simulink model "coursework"  (R2024a)
settings: Solver=FixedStepAuto  StartTime=0.0  StopTime=0.5  FixedStep=0.00001  RelTol=1e-3
values from neighbouring files (symbols this model uses):
  a1 = 80    [PMSM_parameters.m]
  a2 = 200    [PMSM_parameters.m]
  a3 = 360    [PMSM_parameters.m]
  a4 = 520    [PMSM_parameters.m]
  B = 0    [PMSM_parameters.m]
  gamma_lambda = 900000000    [PMSM_parameters.m]
  ia0 = 0    [PMSM_parameters.m]
  ib0 = 0    [PMSM_parameters.m]
  Jm = 60/1000000    (= 6e-05)    [PMSM_parameters.m]
  Ki = 10000    [PMSM_parameters.m]
  Kp = 2000    [PMSM_parameters.m]
  L = 40.03/1000    (= 0.04003)    [PMSM_parameters.m]
  lambda_m = 0.2086    [PMSM_parameters.m]
  np = 5    [PMSM_parameters.m]
  omega0 = 0    [PMSM_parameters.m]
  R = 8.875    [PMSM_parameters.m]
  tao_L = 1    [PMSM_parameters.m]
  theta0 = 0    [PMSM_parameters.m]
  v = 1400    [PMSM_parameters.m]
libraries: dspsrcs4 x1, dspstat3 x1
settings Model: Creator=yuyouyang  LastModifiedBy=yuyouyang

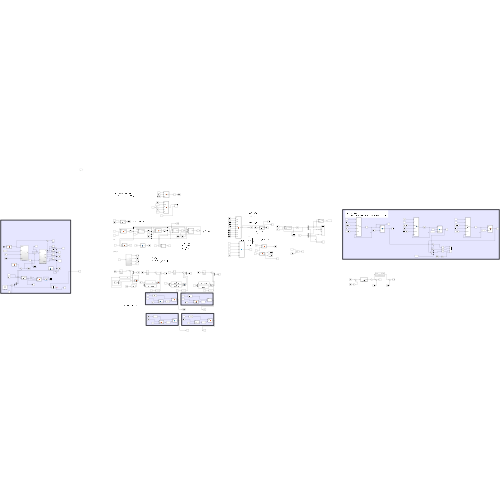
[thumbnail: Simulink's stored preview of the top-level diagram]
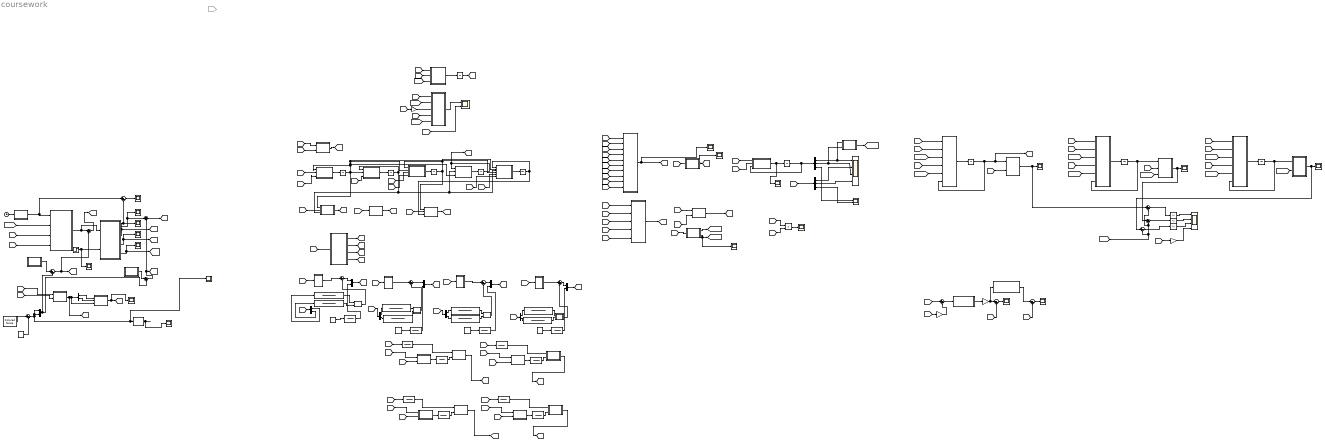
== system coursework ==
  note: Subsystem8
  note: Subsystem7
  note: Subsystem6
  note: Subsystem5
  note: FI_bar & fi_bar
  note: FI & fi
  Abs : Abs  SaturateOnIntegerOverflow=off
  Abs1 : Abs  SaturateOnIntegerOverflow=off
  Abs2 : Abs  SaturateOnIntegerOverflow=off
  Clock2 : Clock
  Colored Noise : dspsrcs4/Colored Noise  Color=pink  InverseFrequencyPower=1  BoundedOutput=on  NumChannels=1  OutputDataType=double  SamplesPerFrame=1  SampleTime=0.01  RandomStream=mt19937ar with seed  Seed=67  SimulateUsing=Interpreted execution
      settings: LibrarySourceBlock=audiosources/Colored Noise
  Constant{,1..3} (4 alike) : Constant  Value=2*v^-1
  Constant4 : Constant  Value=0.1
  Demux10 : Demux  Outputs=3
  Demux{4..7,11} (5 alike) : Demux  Outputs=2
  Demux9 : Demux  Outputs=3
  From71 : From  Commented=on  GotoTag=ym
  Gain : Gain  Gain=2*L
  Gain1 : Gain  Gain=L/R
  Gain2 : Gain  Gain=L
  Gain3 : Gain  Gain=1/np
  Integrator{,1..4,8..10} (8 alike) : Integrator
  Integrator5 : Integrator  InitialCondition=[0;0;0]
  Integrator6 : Integrator  InitialCondition=[0.2086;0]
  MATLAB Function : MATLAB Function  TreatAsAtomicUnit=on
  MATLAB Function1 : MATLAB Function  TreatAsAtomicUnit=on
  MATLAB Function11 : MATLAB Function  TreatAsAtomicUnit=on
  MATLAB Function12 : MATLAB Function  TreatAsAtomicUnit=on
  MATLAB Function13 : MATLAB Function  TreatAsAtomicUnit=on
  MATLAB Function14 : MATLAB Function  TreatAsAtomicUnit=on
  MATLAB Function15 : MATLAB Function  TreatAsAtomicUnit=on
  MATLAB Function16 : MATLAB Function  TreatAsAtomicUnit=on
  MATLAB Function17 : MATLAB Function  TreatAsAtomicUnit=on
  MATLAB Function18 : MATLAB Function  TreatAsAtomicUnit=on
  MATLAB Function19 : MATLAB Function  TreatAsAtomicUnit=on
  MATLAB Function2 : MATLAB Function  TreatAsAtomicUnit=on
  MATLAB Function20 : MATLAB Function  TreatAsAtomicUnit=on
  MATLAB Function21 : MATLAB Function  TreatAsAtomicUnit=on
  MATLAB Function22 : MATLAB Function  TreatAsAtomicUnit=on
  MATLAB Function23 : MATLAB Function  TreatAsAtomicUnit=on
  MATLAB Function24 : MATLAB Function  TreatAsAtomicUnit=on
  MATLAB Function25 : MATLAB Function  TreatAsAtomicUnit=on
  MATLAB Function26 : MATLAB Function  TreatAsAtomicUnit=on
  MATLAB Function27 : MATLAB Function  TreatAsAtomicUnit=on
  MATLAB Function28 : MATLAB Function  TreatAsAtomicUnit=on
  MATLAB Function29 : MATLAB Function  TreatAsAtomicUnit=on
  MATLAB Function3 : MATLAB Function  TreatAsAtomicUnit=on
  MATLAB Function30 : MATLAB Function  TreatAsAtomicUnit=on
  MATLAB Function31 : MATLAB Function  TreatAsAtomicUnit=on
  MATLAB Function32 : MATLAB Function  TreatAsAtomicUnit=on
  MATLAB Function33 : MATLAB Function  TreatAsAtomicUnit=on
  MATLAB Function34 : MATLAB Function  TreatAsAtomicUnit=on
  MATLAB Function35 : MATLAB Function  TreatAsAtomicUnit=on
  MATLAB Function36 : MATLAB Function  TreatAsAtomicUnit=on
  MATLAB Function37 : MATLAB Function  TreatAsAtomicUnit=on
  MATLAB Function38 : MATLAB Function  TreatAsAtomicUnit=on
  MATLAB Function39 : MATLAB Function  TreatAsAtomicUnit=on
  MATLAB Function4 : MATLAB Function  TreatAsAtomicUnit=on
  MATLAB Function40 : MATLAB Function  TreatAsAtomicUnit=on
  MATLAB Function41 : MATLAB Function  TreatAsAtomicUnit=on
  MATLAB Function5 : MATLAB Function  TreatAsAtomicUnit=on
  MATLAB Function6 : MATLAB Function  TreatAsAtomicUnit=on
  MATLAB Function7 : MATLAB Function  TreatAsAtomicUnit=on
  MATLAB Function8 : MATLAB Function  TreatAsAtomicUnit=on
  MATLAB Function9 : MATLAB Function  TreatAsAtomicUnit=on
  Mean : dspstat3/Mean  run=off  InputProcessing=Columns as channels (frame based)  reset_popup=None  directionMode=Each column  dimension=1  roiEnable=off  roiType=Rectangles  roiPortion=Entire ROI  roiOutput=Individual statistics for each ROI  roiFlag=off  roundingMode=Floor  overflowMode=off  outputDataTypeStr=Inherit: Same as accumulator  outputMin=[]  outputMax=[]  outputLastDataTypeStr=Inherit: Same as accumulator
  Mux{1..4,6} (5 alike) : Mux  Inputs=2
  Product : Product
  Scope : Scope  NumInputPorts=4
  Scope{1..2,4,6..9,11,13..16,18} (13 alike) : Scope
  Scope17 : Scope  NumInputPorts=4
  Scope3 : Scope  NumInputPorts=2
  Scope5 : Scope  NumInputPorts=2
  Step4 : Step  Time=0.3  After=tao_L  SampleTime=0
  Subsystem : Subsystem
  Subsystem1 : Subsystem
  Subsystem2 : Subsystem
  Subsystem3 : Subsystem
  Subsystem4 : Subsystem
  Subsystem5 : Subsystem
  Sum{,1..7,11} (9 alike) : Sum  Inputs=|+-
  Sum{9..10,13..15} (5 alike) : Sum  Inputs=|++
  Sum12 : Sum  Inputs=|-+
  Sum8 : Sum  Inputs=|-+
  Surface-Mount PMSM1 : Subsystem
  Transfer Fcn10 : TransferFcn  Denominator=[1 a1]
  Transfer Fcn11 : TransferFcn  Numerator=[a3]  Denominator=[1 2*a3 a3^2]
  Transfer Fcn12 : TransferFcn  Numerator=[a3]  Denominator=[1 a3]
  Transfer Fcn13 : TransferFcn  Denominator=[1 a2]
  Transfer Fcn14 : TransferFcn  Numerator=[a4]  Denominator=[1 2*a4 a4^2]
  Transfer Fcn15 : TransferFcn  Numerator=[a4]  Denominator=[1 a4]
  Transfer Fcn20 : TransferFcn  Numerator=[a1]  Denominator=[1 2*a1 a1^2]
  Transfer Fcn21 : TransferFcn  Numerator=[a2]  Denominator=[1 2*a2 a2^2]
  Transfer Fcn22 : TransferFcn  Numerator=[a3]  Denominator=[1 2*a3 a3^2]
  Transfer Fcn23 : TransferFcn  Numerator=[a4]  Denominator=[1 2*a4 a4^2]
  Transfer Fcn24 : TransferFcn  Numerator=[a2]  Denominator=[1 a2]
  Transfer Fcn25 : TransferFcn  Denominator=[1 a3]
  Transfer Fcn26 : TransferFcn  Numerator=[a3]  Denominator=[1 a3]
  Transfer Fcn27 : TransferFcn  Denominator=[1 a4]
  Transfer Fcn28 : TransferFcn  Numerator=[a4]  Denominator=[1 a4]
  Transfer Fcn4 : TransferFcn  Numerator=[a1]  Denominator=[1 a1]
  Transfer Fcn5 : TransferFcn  Numerator=[a1]  Denominator=[1 2*a1 a1^2]
  Transfer Fcn6 : TransferFcn  Numerator=[a1]  Denominator=[1 a1]
  Transfer Fcn8 : TransferFcn  Numerator=[a2]  Denominator=[1 2*a2 a2^2]
  Transfer Fcn9 : TransferFcn  Numerator=[a2]  Denominator=[1 a2]
  currents iab1 : Scope
  flux lambda_ab3 : Scope
  position estimator : MATLAB Function  TreatAsAtomicUnit=on
  position theta3 : Scope
  speed omega3 : Scope
  speed1 : Scope
  torque load : Scope
  vector control1 : Subsystem
  wires:
  MATLAB Function/1(xi1_dot) -> Integrator/1
  Integrator/1 -> MATLAB Function6/1(xi1), MATLAB Function2/2(xi1), MATLAB Function4/3(xi1), MATLAB Function5/4(xi1), MATLAB Function3/2(xi1), MATLAB Function/1(xi1)  "xi1"
  [i] -> MATLAB Function1/1(i)
  MATLAB Function1/1(ym) -> [ym]
  [i] -> MATLAB Function/3(i)
  [ym] -> MATLAB Function/2(ym)
  MATLAB Function2/1(xi2_dot) -> Integrator1/1
  Integrator1/1 -> MATLAB Function5/3(xi2), MATLAB Function4/2(xi2), MATLAB Function6/3(xi2), MATLAB Function2/1(xi2)  "xi2"
  [ym] -> MATLAB Function2/3(ym)
  MATLAB Function3/1(xi3_dot) -> Integrator2/1
  Integrator2/1 -> MATLAB Function21/1(xi3), MATLAB Function5/2(xi3), MATLAB Function3/1(xi3)  "xi3"
  [ym] -> MATLAB Function3/3(ym)
  [i] -> MATLAB Function3/4(i)
  MATLAB Function4/1(xi4_dot) -> Integrator3/1
  MATLAB Function5/1(xi5_dot) -> Integrator4/1
  Integrator4/1 -> MATLAB Function21/3(xi5), MATLAB Function5/1(xi5)  "xi5"
  [i] -> MATLAB Function5/5(i)
  [ym] -> MATLAB Function5/6(ym)
  [i] -> MATLAB Function6/2(i)
  MATLAB Function6/1(FI) -> [FI]
  MATLAB Function7/1(fi) -> [fi]
  Sum/1 -> Mux1/1
  Constant/1 -> Transfer Fcn6/1
  Mux1/1 -> [fi_bar1]
  Constant1/1 -> Transfer Fcn9/1
  Sum1/1 -> Mux2/1
  Mux2/1 -> [fi_bar2]
  Mux3/1 -> [fi_bar3]
  Sum2/1 -> Mux3/1
  Constant2/1 -> Transfer Fcn12/1
  Mux4/1 -> [fi_bar4]
  Sum3/1 -> Mux4/1
  Constant3/1 -> Transfer Fcn15/1
  Integrator3/1 -> [xi4], MATLAB Function4/1(xi4)  "xi4"
  [FI] -> Demux4/1
  Demux4/1 -> Transfer Fcn5/1
  Demux4/2 -> Transfer Fcn20/1
  Transfer Fcn5/1 -> MATLAB Function12/1(u)
  Transfer Fcn20/1 -> MATLAB Function12/2(z)
  MATLAB Function12/1(y) -> Sum/2
  [FI] -> Demux5/1
  Demux5/1 -> Transfer Fcn8/1
  Demux5/2 -> Transfer Fcn21/1
  Transfer Fcn8/1 -> MATLAB Function13/1(u)
  Transfer Fcn21/1 -> MATLAB Function13/2(z)
  MATLAB Function13/1(y) -> Sum1/2
  [FI] -> Demux6/1
  Demux6/1 -> Transfer Fcn11/1
  Demux6/2 -> Transfer Fcn22/1
  Transfer Fcn11/1 -> MATLAB Function14/1(u)
  Transfer Fcn22/1 -> MATLAB Function14/2(z)
  MATLAB Function14/1(y) -> Sum2/2
  [FI] -> Demux7/1
  Demux7/1 -> Transfer Fcn14/1
  Demux7/2 -> Transfer Fcn23/1
  Transfer Fcn14/1 -> MATLAB Function15/1(u)
  Transfer Fcn23/1 -> MATLAB Function15/2(z)
  MATLAB Function15/1(y) -> Sum3/2
  Subsystem1/1(y) -> Sum3/1
  Subsystem2/1(y) -> Sum2/1
  Subsystem3/1(y) -> Sum1/1
  Subsystem4/1(y) -> Sum/1
  [FI] -> MATLAB Function16/1(FI)
  [FI_bar1] -> MATLAB Function16/2(FI_bar1)
  [FI_bar2] -> MATLAB Function16/3(FI_bar2)
  [FI_bar3] -> MATLAB Function16/4(FI_bar3)
  [FI_bar4] -> MATLAB Function16/5(FI_bar4)
  [fi] -> MATLAB Function16/6(fi)
  [fi_bar1] -> MATLAB Function16/7(fi_bar1)
  [fi_bar4] -> MATLAB Function16/10(fi_bar4)
  [fi_bar3] -> MATLAB Function16/9(fi_bar3)
  [fi_bar2] -> MATLAB Function16/8(fi_bar2)
  MATLAB Function16/1(M) -> Scope13/1, [M]  "M(t)"
  [M] -> MATLAB Function17/1(M)
  MATLAB Function17/1(delta) -> Scope11/1, [delta]
  MATLAB Function20/1(eta_hat_dot) -> Scope2/1, Integrator5/1
  Integrator5/1 -> MATLAB Function20/3(eta_hat), Demux9/1  "eta_hat"
  [Y_eta] -> MATLAB Function20/2(Y_eta)
  [delta] -> MATLAB Function20/1(delta)
  [eta] -> Demux10/1
  Demux9/1 -> MATLAB Function35/1(etam1), Scope/1  "eta_hat1"
  Demux10/1 -> Scope/2  "eta1"
  Demux9/2 -> MATLAB Function35/2(etam2), Scope/3  "eta_hat2"
  Demux10/2 -> Scope/4  "eta2"
  Demux9/3 -> Scope3/1  "eta_hat3"
  Demux10/3 -> Scope3/2  "eta3"
  [bv] -> MATLAB Function23/2(bv)
  [bi] -> MATLAB Function23/1(bi)
  Demux11/1 -> MATLAB Function24/1(eta1)
  MATLAB Function23/1(eta_m) -> [eta_m], MATLAB Function24/3(eta_m), Demux11/1
  Demux11/2 -> MATLAB Function24/2(eta2)
  MATLAB Function24/1(eta) -> Scope1/1, [eta]
  Clock2/1 -> MATLAB Function25/1(u)
  Surface-Mount PMSM1/4(lambda_ab) -> flux lambda_ab3/1, [lambda_ab]
  MATLAB Function25/1(y) -> vector control1/1(speed ref), Sum7/1
  Surface-Mount PMSM1/1(iab) -> Sum10/1, currents iab1/1
  Surface-Mount PMSM1/2(omega) -> [omega], Sum7/2, speed omega3/1
  Step4/1 -> torque load/1, Surface-Mount PMSM1/2(tau_L)
  Surface-Mount PMSM1/3(theta) -> position theta3/1, [theta]
  [i] -> vector control1/3(Iab)
  Sum7/1 -> speed1/1
  [theta] -> vector control1/2(theta)
  [omega] -> vector control1/4(omega)
  vector control1/1(Vab) -> Surface-Mount PMSM1/1(vab), Sum9/1
  Sum10/1 -> [i]
  [xi4] -> MATLAB Function7/1(xi4)
  [xi4] -> Subsystem4/1(xi4)
  [xi4] -> Subsystem3/1(xi4)
  [xi4] -> Subsystem2/1(xi4)
  [xi4] -> Subsystem1/1(xi4)
  Sum9/1 -> [V]
  [i] -> MATLAB Function21/2(i)
  MATLAB Function21/1(y) -> [y]
  MATLAB Function37/1(y) -> Sum13/1
  MATLAB Function29/1(z) -> [z2]
  MATLAB Function31/1(z) -> [z3]
  MATLAB Function33/1(z) -> [z4]
  [y] -> MATLAB Function18/1(y)
  [z1] -> MATLAB Function18/2(z1)
  [z2] -> MATLAB Function18/3(z2)
  [z3] -> MATLAB Function18/4(z3)
  [z4] -> MATLAB Function18/5(z4)
  MATLAB Function18/1(Z) -> [Z]
  [M] -> MATLAB Function19/1(M)
  [Z] -> MATLAB Function19/2(Z)
  MATLAB Function19/1(Y) -> [Y]
  [Y] -> MATLAB Function22/1(u)
  MATLAB Function22/1(Y_lambda) -> [Y_lambda]
  MATLAB Function22/2(Y_eta) -> Scope8/1, [Y_eta]
  [delta] -> Product/1
  [eta] -> Product/2
  Product/1 -> Scope6/1
  Transfer Fcn6/1 -> Mux1/2
  Transfer Fcn9/1 -> Mux2/2
  Transfer Fcn12/1 -> Mux3/2
  Transfer Fcn15/1 -> Mux4/2
  MATLAB Function27/1(z) -> [z1]
  MATLAB Function26/1(y) -> Transfer Fcn10/1
  [y] -> Transfer Fcn4/1
  Transfer Fcn4/1 -> MATLAB Function27/1(y_filter)
  [FI_bar1] -> MATLAB Function26/2(FI_filter)
  Transfer Fcn10/1 -> MATLAB Function27/2(p)
  [ym] -> MATLAB Function26/1(ym)
  [y] -> Transfer Fcn24/1
  Transfer Fcn13/1 -> MATLAB Function29/2(p)
  [ym] -> MATLAB Function28/1(ym)
  Transfer Fcn24/1 -> MATLAB Function29/1(y_filter)
  MATLAB Function28/1(y) -> Transfer Fcn13/1
  [FI_bar2] -> MATLAB Function28/2(FI_filter)
  [y] -> Transfer Fcn26/1
  [ym] -> MATLAB Function30/1(ym)
  Transfer Fcn25/1 -> MATLAB Function31/2(p)
  Transfer Fcn26/1 -> MATLAB Function31/1(y_filter)
  MATLAB Function30/1(y) -> Transfer Fcn25/1
  [FI_bar3] -> MATLAB Function30/2(FI_filter)
  [y] -> Transfer Fcn28/1
  Transfer Fcn28/1 -> MATLAB Function33/1(y_filter)
  [ym] -> MATLAB Function32/1(ym)
  Transfer Fcn27/1 -> MATLAB Function33/2(p)
  MATLAB Function32/1(y) -> Transfer Fcn27/1
  [FI_bar4] -> MATLAB Function32/2(FI_filter)
  [FI] -> Subsystem/1(In1)
  Subsystem/1(y) -> [FI_bar1]
  Subsystem/2(y1) -> [FI_bar2]
  Subsystem/3(y2) -> [FI_bar3]
  Subsystem/4(y3) -> [FI_bar4]
  MATLAB Function8/1(lambda_dot) -> Integrator6/1
  [i] -> MATLAB Function8/1(i)
  [V] -> MATLAB Function8/2(v)
  [eta_m] -> MATLAB Function8/3(eta_m)
  Integrator6/1 -> [lambda]
  [FI] -> MATLAB Function9/1(FI)
  [lambda] -> MATLAB Function9/2(lambda)
  [eta] -> MATLAB Function9/5(eta)
  [fi] -> MATLAB Function9/4(fi)
  [bi] -> Gain/1
  Gain/1 -> MATLAB Function9/3(eta1)
  MATLAB Function9/1(y) -> Scope5/1
  [y] -> Scope5/2
  [V] -> MATLAB Function1/2(v)
  MATLAB Function35/1(etam) -> [etam_hat]
  MATLAB Function11/1(chi1_dot) -> Integrator8/1
  Integrator8/1 -> [chi], MATLAB Function36/1(chi1), MATLAB Function11/6(chi1)  "chi1"
  [Y_lambda] -> MATLAB Function11/5(Y_lambda)
  [delta] -> MATLAB Function11/4(delta)
  [etam_hat] -> MATLAB Function11/3(etam_hat)
  [V] -> MATLAB Function11/2(v)
  [i] -> MATLAB Function11/1(i)
  [bi] -> MATLAB Function36/2(bi)
  MATLAB Function36/1(lambda_hat) -> Sum4/1, Scope14/1  "14"
  [i] -> MATLAB Function38/1(i)
  Integrator9/1 -> MATLAB Function39/1(chi1), MATLAB Function38/6(chi1)  "chi1"
  [Y_lambda] -> MATLAB Function38/5(Y_lambda)
  MATLAB Function38/1(chi2_dot) -> Integrator9/1
  [etam_hat] -> MATLAB Function38/3(etam_hat)
  [V] -> MATLAB Function38/2(v)
  [delta] -> MATLAB Function38/4(delta)
  [bv] -> MATLAB Function39/2(bv)
  [etam_hat] -> MATLAB Function39/3(etam_hat)
  MATLAB Function39/1(lambda_hat) -> Sum5/1, Scope15/1  "15"
  MATLAB Function40/1(chi2_dot) -> Integrator10/1
  [etam_hat] -> MATLAB Function41/2(etam_hat)
  [delta] -> MATLAB Function40/4(delta)
  [i] -> MATLAB Function40/1(i)
  [Y_lambda] -> MATLAB Function40/5(Y_lambda)
  [V] -> MATLAB Function40/2(v)
  [etam_hat] -> MATLAB Function40/3(etam_hat)
  MATLAB Function41/1(lambda_hat) -> Sum6/1, Scope16/1  "16"
  Integrator10/1 -> MATLAB Function40/6(chi1), MATLAB Function41/1(chi1)  "chi1"
  [lambda_ab] -> Sum6/2, Sum5/2, Sum4/2
  Sum4/1 -> Abs/1
  Sum5/1 -> Abs1/1
  Sum6/1 -> Abs2/1
  Abs/1 -> Scope17/1
  Abs1/1 -> Scope17/2
  Abs2/1 -> Scope17/3
  [bv] -> Gain1/1
  Gain1/1 -> Scope17/4
  [theta] -> Sum8/2
  Sum8/1 -> Scope18/1
  [i] -> Gain2/1
  Gain2/1 -> Sum11/2
  [chi] -> Sum11/1
  Sum11/1 -> position estimator/1(x)
  position estimator/1(hat_theta) -> Gain3/1
  Gain3/1 -> Subsystem5/1(hat_theta), Sum8/1
  Subsystem5/1(hat_omega) -> Sum12/1
  [omega] -> Sum12/2
  Sum12/1 -> Scope4/1
  Sum13/1 -> [bv], Sum9/2
  MATLAB Function34/1(y) -> Sum14/1
  Mux6/1 -> Sum14/2, Sum13/2
  Sum14/1 -> Sum10/2, [bi]
  Mean/1 -> Scope9/1
  Colored Noise/1 -> Sum15/1
  Constant4/1 -> Sum15/2
  Sum15/1 -> Scope7/1, Mean/1, Mux6/2, Mux6/1

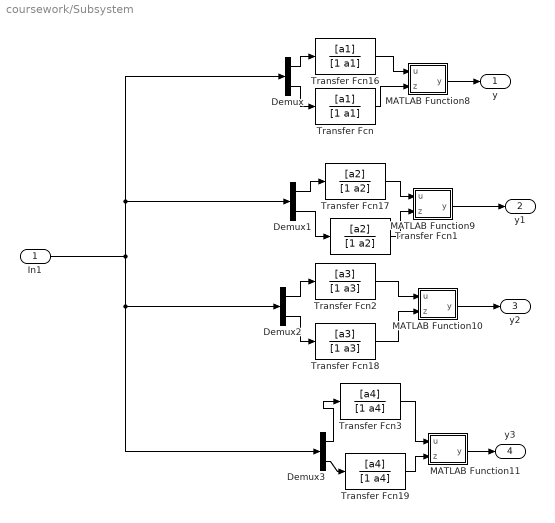
== system coursework/Subsystem ==
  In1 : Inport
  Demux{,1..3} (4 alike) : Demux  Outputs=2
  MATLAB Function10 : MATLAB Function  TreatAsAtomicUnit=on
  MATLAB Function11 : MATLAB Function  TreatAsAtomicUnit=on
  MATLAB Function8 : MATLAB Function  TreatAsAtomicUnit=on
  MATLAB Function9 : MATLAB Function  TreatAsAtomicUnit=on
  Transfer Fcn : TransferFcn  Numerator=[a1]  Denominator=[1 a1]
  Transfer Fcn1 : TransferFcn  Numerator=[a2]  Denominator=[1 a2]
  Transfer Fcn16 : TransferFcn  Numerator=[a1]  Denominator=[1 a1]
  Transfer Fcn17 : TransferFcn  Numerator=[a2]  Denominator=[1 a2]
  Transfer Fcn18 : TransferFcn  Numerator=[a3]  Denominator=[1 a3]
  Transfer Fcn19 : TransferFcn  Numerator=[a4]  Denominator=[1 a4]
  Transfer Fcn2 : TransferFcn  Numerator=[a3]  Denominator=[1 a3]
  Transfer Fcn3 : TransferFcn  Numerator=[a4]  Denominator=[1 a4]
  y : Outport
  y1 : Outport  Port=2
  y2 : Outport  Port=3
  y3 : Outport  Port=4
  wires:
  MATLAB Function10/1(y) -> y2/1
  Transfer Fcn17/1 -> MATLAB Function9/1(u)
  Transfer Fcn18/1 -> MATLAB Function10/2(z)
  Transfer Fcn16/1 -> MATLAB Function8/1(u)
  In1/1 -> Demux2/1, Demux3/1, Demux1/1, Demux/1
  MATLAB Function9/1(y) -> y1/1
  Transfer Fcn/1 -> MATLAB Function8/2(z)
  Transfer Fcn2/1 -> MATLAB Function10/1(u)
  Demux/1 -> Transfer Fcn16/1
  Demux3/1 -> Transfer Fcn3/1
  Transfer Fcn19/1 -> MATLAB Function11/2(z)
  Transfer Fcn3/1 -> MATLAB Function11/1(u)
  Demux2/2 -> Transfer Fcn18/1
  Demux1/2 -> Transfer Fcn1/1
  Demux/2 -> Transfer Fcn/1
  MATLAB Function8/1(y) -> y/1
  Demux3/2 -> Transfer Fcn19/1
  Demux2/1 -> Transfer Fcn2/1
  Transfer Fcn1/1 -> MATLAB Function9/2(z)
  Demux1/1 -> Transfer Fcn17/1
  MATLAB Function11/1(y) -> y3/1

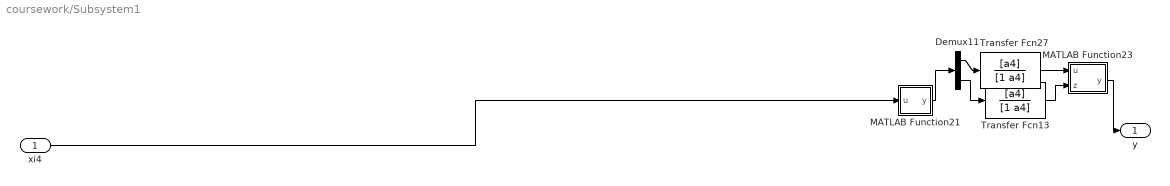
== system coursework/Subsystem1 ==
  xi4 : Inport
  Demux11 : Demux  Outputs=2
  MATLAB Function21 : MATLAB Function  TreatAsAtomicUnit=on
  MATLAB Function23 : MATLAB Function  TreatAsAtomicUnit=on
  Transfer Fcn13 : TransferFcn  Numerator=[a4]  Denominator=[1 a4]
  Transfer Fcn27 : TransferFcn  Numerator=[a4]  Denominator=[1 a4]
  y : Outport
  wires:
  MATLAB Function21/1(y) -> Demux11/1
  Transfer Fcn27/1 -> MATLAB Function23/1(u)
  Demux11/2 -> Transfer Fcn13/1
  xi4/1 -> MATLAB Function21/1(u)
  Demux11/1 -> Transfer Fcn27/1
  MATLAB Function23/1(y) -> y/1
  Transfer Fcn13/1 -> MATLAB Function23/2(z)

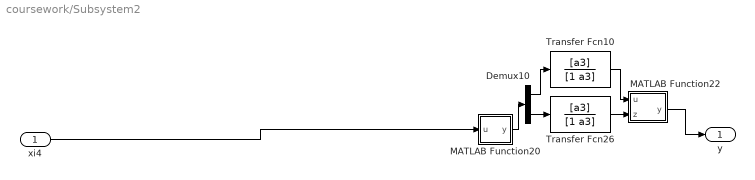
== system coursework/Subsystem2 ==
  xi4 : Inport
  Demux10 : Demux  Outputs=2
  MATLAB Function20 : MATLAB Function  TreatAsAtomicUnit=on
  MATLAB Function22 : MATLAB Function  TreatAsAtomicUnit=on
  Transfer Fcn10 : TransferFcn  Numerator=[a3]  Denominator=[1 a3]
  Transfer Fcn26 : TransferFcn  Numerator=[a3]  Denominator=[1 a3]
  y : Outport
  wires:
  xi4/1 -> MATLAB Function20/1(u)
  MATLAB Function22/1(y) -> y/1
  Transfer Fcn26/1 -> MATLAB Function22/2(z)
  MATLAB Function20/1(y) -> Demux10/1
  Transfer Fcn10/1 -> MATLAB Function22/1(u)
  Demux10/2 -> Transfer Fcn26/1
  Demux10/1 -> Transfer Fcn10/1

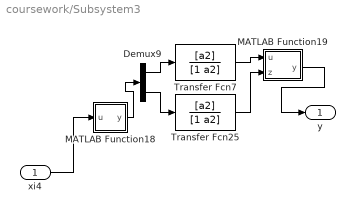
== system coursework/Subsystem3 ==
  xi4 : Inport
  Demux9 : Demux  Outputs=2
  MATLAB Function18 : MATLAB Function  TreatAsAtomicUnit=on
  MATLAB Function19 : MATLAB Function  TreatAsAtomicUnit=on
  Transfer Fcn25 : TransferFcn  Numerator=[a2]  Denominator=[1 a2]
  Transfer Fcn7 : TransferFcn  Numerator=[a2]  Denominator=[1 a2]
  y : Outport
  wires:
  MATLAB Function19/1(y) -> y/1
  xi4/1 -> MATLAB Function18/1(u)
  Demux9/1 -> Transfer Fcn7/1
  Transfer Fcn7/1 -> MATLAB Function19/1(u)
  Demux9/2 -> Transfer Fcn25/1
  Transfer Fcn25/1 -> MATLAB Function19/2(z)
  MATLAB Function18/1(y) -> Demux9/1

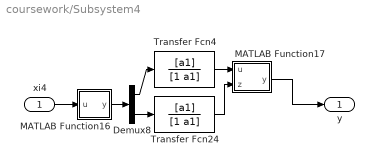
== system coursework/Subsystem4 ==
  xi4 : Inport
  Demux8 : Demux  Outputs=2
  MATLAB Function16 : MATLAB Function  TreatAsAtomicUnit=on
  MATLAB Function17 : MATLAB Function  TreatAsAtomicUnit=on
  Transfer Fcn24 : TransferFcn  Numerator=[a1]  Denominator=[1 a1]
  Transfer Fcn4 : TransferFcn  Numerator=[a1]  Denominator=[1 a1]
  y : Outport
  wires:
  xi4/1 -> MATLAB Function16/1(u)
  Transfer Fcn24/1 -> MATLAB Function17/2(z)
  Transfer Fcn4/1 -> MATLAB Function17/1(u)
  Demux8/1 -> Transfer Fcn4/1
  Demux8/2 -> Transfer Fcn24/1
  MATLAB Function17/1(y) -> y/1
  MATLAB Function16/1(y) -> Demux8/1

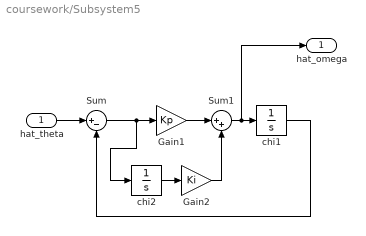
== system coursework/Subsystem5 ==
  hat_theta : Inport
  Gain1 : Gain  Gain=Kp
  Gain2 : Gain  Gain=Ki
  Sum : Sum  Inputs=|+-
  Sum1 : Sum  Inputs=|++
  chi1 : Integrator
  chi2 : Integrator
  hat_omega : Outport
  wires:
  Gain2/1 -> Sum1/2
  hat_theta/1 -> Sum/1
  Gain1/1 -> Sum1/1
  chi1/1 -> Sum/2
  chi2/1 -> Gain2/1
  Sum1/1 -> hat_omega/1, chi1/1
  Sum/1 -> chi2/1, Gain1/1

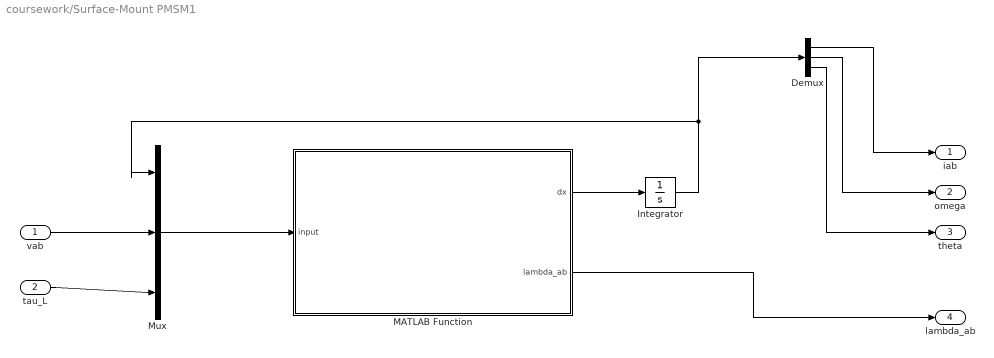
== system coursework/Surface-Mount PMSM1 ==
  vab : Inport
  tau_L : Inport  Port=2
  Demux : Demux  Outputs=3
  Integrator : Integrator  InitialCondition=[ia0; ib0; omega0; theta0]
  MATLAB Function : MATLAB Function  TreatAsAtomicUnit=on
  Mux : Mux  Inputs=3
  iab : Outport
  omega : Outport  Port=2
  theta : Outport  Port=3
  lambda_ab : Outport  Port=4
  wires:
  Demux/2 -> omega/1
  Demux/1 -> iab/1
  Integrator/1 -> Demux/1, Mux/1
  vab/1 -> Mux/2
  Mux/1 -> MATLAB Function/1(input)
  tau_L/1 -> Mux/3
  MATLAB Function/2(lambda_ab) -> lambda_ab/1
  MATLAB Function/1(dx) -> Integrator/1
  Demux/3 -> theta/1

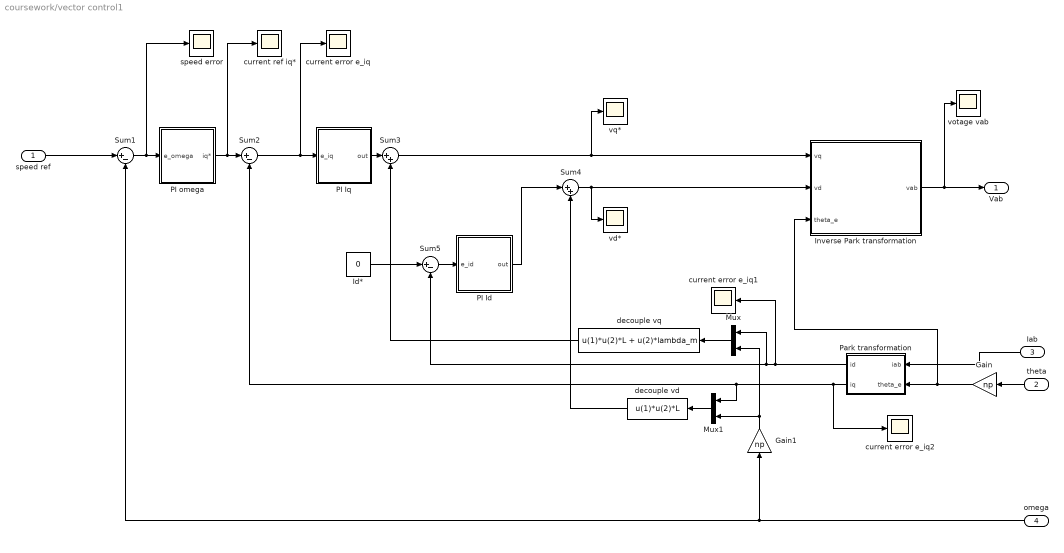
== system coursework/vector control1 ==
  speed ref : Inport
  theta : Inport  Port=2
  Iab : Inport  Port=3
  omega : Inport  Port=4
  Gain : Gain  Gain=np
  Gain1 : Gain  Gain=np
  Id* : Constant  Value=0
  Inverse Park transformation : MATLAB Function  TreatAsAtomicUnit=on
  Mux : Mux  Inputs=2
  Mux1 : Mux  Inputs=2
  PI Id : Subsystem
  PI Iq : Subsystem
  PI omega : Subsystem
  Park transformation : MATLAB Function  TreatAsAtomicUnit=on
  Sum1 : Sum  Inputs=|+-
  Sum2 : Sum  Inputs=|+-
  Sum3 : Sum  Inputs=|++
  Sum4 : Sum  Inputs=|++
  Sum5 : Sum  Inputs=|+-
  current error e_iq : Scope
  current error e_iq1 : Scope
  current error e_iq2 : Scope
  current ref iq* : Scope
  decouple vd : Fcn  Expr=u(1)*u(2)*L
  decouple vq : Fcn  Expr=u(1)*u(2)*L + u(2)*lambda_m
  speed error : Scope
  vd* : Scope
  votage vab : Scope
  vq* : Scope
  Vab : Outport
  wires:
  speed ref/1 -> Sum1/1
  Id*/1 -> Sum5/1
  Iab/1 -> Park transformation/1(iab)
  PI Id/1(out) -> Sum4/1
  Park transformation/2(iq) -> Mux1/1, Sum2/2, current error e_iq2/1
  omega/1 -> Sum1/2, Gain1/1
  decouple vd/1 -> Sum4/2
  decouple vq/1 -> Sum3/2
  Sum5/1 -> PI Id/1(e_id)
  Mux1/1 -> decouple vd/1
  Sum4/1 -> vd*/1, Inverse Park transformation/2(vd)
  Park transformation/1(id) -> current error e_iq1/1, Mux/1, Sum5/2
  Sum1/1 -> speed error/1, PI omega/1(e_omega)
  Sum2/1 -> current error e_iq/1, PI Iq/1(e_iq)
  Gain/1 -> Inverse Park transformation/3(theta_e), Park transformation/2(theta_e)
  Gain1/1 -> Mux1/2, Mux/2
  Inverse Park transformation/1(vab) -> Vab/1, votage vab/1
  Sum3/1 -> vq*/1, Inverse Park transformation/1(vq)
  Mux/1 -> decouple vq/1
  PI omega/1(iq*) -> current ref iq*/1, Sum2/1
  PI Iq/1(out) -> Sum3/1
  theta/1 -> Gain/1

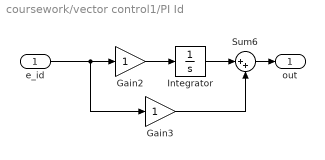
== system coursework/vector control1/PI Id ==
  e_id : Inport
  Gain2 : Gain
  Gain3 : Gain
  Integrator : Integrator
  Sum6 : Sum  Inputs=|++
  out : Outport
  wires:
  Integrator/1 -> Sum6/1
  Gain3/1 -> Sum6/2
  e_id/1 -> Gain3/1, Gain2/1
  Gain2/1 -> Integrator/1
  Sum6/1 -> out/1

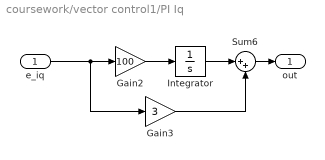
== system coursework/vector control1/PI Iq ==
  e_iq : Inport
  Gain2 : Gain  Gain=100
  Gain3 : Gain  Gain=3
  Integrator : Integrator
  Sum6 : Sum  Inputs=|++
  out : Outport
  wires:
  Integrator/1 -> Sum6/1
  Gain3/1 -> Sum6/2
  e_iq/1 -> Gain3/1, Gain2/1
  Gain2/1 -> Integrator/1
  Sum6/1 -> out/1

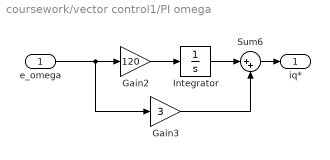
== system coursework/vector control1/PI omega ==
  e_omega : Inport
  Gain2 : Gain  Gain=120
  Gain3 : Gain  Gain=3
  Integrator : Integrator
  Sum6 : Sum  Inputs=|++
  iq* : Outport
  wires:
  Integrator/1 -> Sum6/1
  Gain3/1 -> Sum6/2
  e_omega/1 -> Gain3/1, Gain2/1
  Gain2/1 -> Integrator/1
  Sum6/1 -> iq*/1

== matlab function coursework/MATLAB Function7 ==
  data: xi4 input; fi output; v parameter
function fi = fcn(xi4,v)

fi = [2*xi4;2*v^-1];

== matlab function coursework/Subsystem/MATLAB Function8 ==
  data: u input; y output; z input
function y = fcn(u,z)

y = [u;z];

== matlab function coursework/Subsystem/MATLAB Function9 ==
  data: u input; y output; z input
function y = fcn(u,z)

y = [u;z];

== matlab function coursework/Subsystem/MATLAB Function10 ==
  data: u input; y output; z input
function y = fcn(u,z)

y = [u;z];

== matlab function coursework/Subsystem/MATLAB Function11 ==
  data: u input; y output; z input
function y = fcn(u,z)

y = [u;z];

== matlab function coursework/MATLAB Function12 ==
  data: u input; y output; z input
function y = fcn(u,z)

y = [u;z];

== matlab function coursework/MATLAB Function13 ==
  data: u input; y output; z input
function y = fcn(u,z)

y = [u;z];

== matlab function coursework/MATLAB Function14 ==
  data: u input; y output; z input
function y = fcn(u,z)

y = [u;z];

== matlab function coursework/MATLAB Function15 ==
  data: u input; y output; z input
function y = fcn(u,z)

y = [u;z];

== matlab function coursework/MATLAB Function ==
  data: xi1 input; xi1_dot output; ym input; i input; L parameter; v parameter
function xi1_dot = fcn(xi1,ym,i, L, v)

xi1_dot = -v*xi1+2*v*ym+2*v^2*L*i;

== matlab function coursework/Subsystem4/MATLAB Function16 ==
  data: u input; y output
function y = fcn(u)

y = 2*u;

== matlab function coursework/Subsystem4/MATLAB Function17 ==
  data: u input; y output; z input
function y = fcn(u,z)

y = [u;z];

== matlab function coursework/Subsystem3/MATLAB Function18 ==
  data: u input; y output
function y = fcn(u)

y = 2*u;

== matlab function coursework/Subsystem3/MATLAB Function19 ==
  data: u input; y output; z input
function y = fcn(u,z)

y = [u;z];

== matlab function coursework/Subsystem2/MATLAB Function20 ==
  data: u input; y output
function y = fcn(u)

y = 2*u;

== matlab function coursework/Subsystem1/MATLAB Function21 ==
  data: u input; y output
function y = fcn(u)

y = 2*u;

== matlab function coursework/Subsystem2/MATLAB Function22 ==
  data: u input; y output; z input
function y = fcn(u,z)

y = [u;z];

== matlab function coursework/Subsystem1/MATLAB Function23 ==
  data: u input; y output; z input
function y = fcn(u,z)

y = [u;z];

== matlab function coursework/MATLAB Function16 ==
  data: FI input; M output; FI_bar1 input; FI_bar2 input; FI_bar3 input; FI_bar4 input; fi input; fi_bar1 input; fi_bar2 input; fi_bar3 input; fi_bar4 input
function M = fcn(FI,FI_bar1,FI_bar2,FI_bar3,FI_bar4,fi,fi_bar1,fi_bar2,fi_bar3,fi_bar4)

M = [FI' fi';FI_bar1' fi_bar1';FI_bar2' fi_bar2';FI_bar3' fi_bar3';FI_bar4' fi_bar4'];

== matlab function coursework/MATLAB Function17 ==
  data: M input; delta output
function delta = fcn(M)

delta = det(M);

== matlab function coursework/MATLAB Function37 ==
  data: y output
function y = fcn()

y = [0.2;-0.1];

== matlab function coursework/MATLAB Function8 ==
  data: i input; lambda_dot output; v input; eta_m input; R parameter
function lambda_dot = fcn(i,v,eta_m,R)

lambda_dot = -R*i+v+eta_m;

== matlab function coursework/MATLAB Function9 ==
  data: FI input; y output; lambda input; eta1 input; fi input; eta input
function y = fcn(FI,lambda,eta1,fi,eta)

y = FI'*(lambda+1/2*eta1)+fi'*eta;

== matlab function coursework/MATLAB Function34 ==
  data: y output
function y = fcn()

y = [0.4;-0.3];

== matlab function coursework/MATLAB Function20 ==
  data: delta input; eta_hat_dot output; Y_eta input; eta_hat input; gamma_eta parameter
function eta_hat_dot = fcn(delta,Y_eta,eta_hat,gamma_eta)

eta_hat_dot = 90000000000*gamma_eta*delta*(Y_eta-delta*eta_hat);

== matlab function coursework/MATLAB Function21 ==
  data: xi3 input; y output; i input; xi5 input; v parameter; L parameter
function y = fcn(xi3,i,xi5, v, L)

y = xi3-v*L^2*i'*i-xi5;

== matlab function coursework/MATLAB Function26 ==
  data: ym input; y output; FI_filter input
function y = fcn(ym,FI_filter)

y = ym'*FI_filter;

== matlab function coursework/MATLAB Function27 ==
  data: y_filter input; z output; p input
function z = fcn(y_filter,p)

z = y_filter+p;

== matlab function coursework/MATLAB Function28 ==
  data: ym input; y output; FI_filter input
function y = fcn(ym,FI_filter)

y = ym'*FI_filter;

== matlab function coursework/MATLAB Function29 ==
  data: y_filter input; z output; p input
function z = fcn(y_filter,p)

z = y_filter+p;

== matlab function coursework/Surface-Mount PMSM1/MATLAB Function ==
  data: input input; dx output; lambda_ab output; R parameter; L parameter; lambda_m parameter; np parameter; Jm parameter; B parameter
function [dx, lambda_ab] = fcn (input, R, L, lambda_m, np, Jm, B)
%#codegen

%%%%%inputs %%%%%
ia=input(1) ;
ib=input(2) ;
iab= [ia; ib];
omega=input(3) ;
theta=input(4) ;
va=input(5) ;
vb=input(6) ;
vab= [va; vb];
tau_L = input(7);

%%%%%denotations%%%%%%
C= [cos(np*theta) ; sin(np*theta)];
J=[0, -1;1,0];
dC=np*J*C;


%%%%%%%%%5 Dynamic model %%%%%%%
%%% Non-salient Permanent Magnet Synchronous Machines %%%
dot_iab= (1/L) * (-R*iab-omega*lambda_m*dC + vab) ;
dot_omega= (1/Jm) * (-B*omega + lambda_m*iab'*dC-tau_L);
dot_theta=omega;
lambda_ab=L*iab+lambda_m*C;

%%%%%%%%%%%%%%

dx= [dot_iab; dot_omega; dot_theta];

== matlab function coursework/MATLAB Function1 ==
  data: ym output; i input; R parameter; v input
function ym = fcn(i,R, v)

ym = -R*i+v;

== matlab function coursework/vector control1/Inverse Park transformation ==
  data: vq input; vab output; vd input; theta_e input
function vab = fcn(vq, vd, theta_e)


va=vd*cos(theta_e)-vq*sin(theta_e);
vb=vd*sin(theta_e)+vq*cos(theta_e);
vab=[va;vb];

== matlab function coursework/vector control1/Park transformation ==
  data: iab input size=2*1; id output size=1*1; theta_e input; iq output
function [id,iq] = fcn(iab, theta_e)

ia=iab(1);
ib=iab(2);
id=ia*cos(theta_e)+ib*sin(theta_e);
iq=-ia*sin(theta_e)+ib*cos(theta_e);

== matlab function coursework/MATLAB Function23 ==
  data: bi input; eta_m output; bv input; R parameter
function eta_m = fcn(bi,bv,R)

eta_m = R*bi-bv;

== matlab function coursework/MATLAB Function24 ==
  data: eta1 input; eta output; eta2 input; eta_m input
function eta = fcn(eta1,eta2,eta_m)

eta = [eta1 eta2 eta_m'*eta_m]';

== matlab function coursework/MATLAB Function25 ==
  data: u input; y output
function y = fcn(u)
if u >= 0 && u <= 0.2
        y = 2615 * u;
    elseif u > 0.2 && u <= 1
        y = 523;
    else
        y = -1;
    end

== matlab function coursework/MATLAB Function30 ==
  data: ym input; y output; FI_filter input
function y = fcn(ym,FI_filter)

y = ym'*FI_filter;

== matlab function coursework/MATLAB Function31 ==
  data: y_filter input; z output; p input
function z = fcn(y_filter,p)

z = y_filter+p;

== matlab function coursework/MATLAB Function32 ==
  data: ym input; y output; FI_filter input
function y = fcn(ym,FI_filter)

y = ym'*FI_filter;

== matlab function coursework/MATLAB Function33 ==
  data: y_filter input; z output; p input
function z = fcn(y_filter,p)

z = y_filter+p;

== matlab function coursework/MATLAB Function18 ==
  data: y input; Z output; z1 input; z2 input; z3 input; z4 input
function Z = fcn(y,z1,z2,z3,z4)

Z =[y;z1;z2;z3;z4];

== matlab function coursework/MATLAB Function2 ==
  data: xi2 input; xi1 input; ym input; xi2_dot output; v parameter
function xi2_dot = fcn(xi2,xi1,ym,v)

xi2_dot = -v*xi2+xi1+2*ym;

== matlab function coursework/MATLAB Function19 ==
  data: M input; Y output; Z input
function Y  = fcn(M,Z)
Y=det(M)*pinv(M)*Z;

% ce=poly(M);
% cesize=max(size(ce));
% p=[0 ce(1:(cesize-1))];
% s = (-1)^(max(size(M))+1);
% B = s*polyvalm(p,M);
% Y=B*Z;

== matlab function coursework/MATLAB Function22 ==
  data: u input; Y_lambda output; Y_eta output
function [Y_lambda,Y_eta] = fcn(u)

Y_lambda =[u(1);u(2)];
Y_eta = [u(3);u(4);u(5)];

== matlab function coursework/MATLAB Function11 ==
  data: chi1_dot output; i input; v input; etam_hat input; delta input; Y_lambda input; chi1 input; R parameter; gamma_lambda parameter
function chi1_dot = fcn(i,v,etam_hat,delta,Y_lambda,chi1, R, gamma_lambda)

chi1_dot = -R*i+v+etam_hat+gamma_lambda*delta*(Y_lambda-delta*chi1);

== matlab function coursework/MATLAB Function35 ==
  data: etam1 input; etam output; etam2 input
function etam = fcn(etam1,etam2)

etam = [etam1;etam2];

== matlab function coursework/MATLAB Function36 ==
  data: chi1 input; lambda_hat output; bi input; L parameter
function lambda_hat = fcn(chi1,bi,L)

lambda_hat = chi1-L*bi;

== matlab function coursework/MATLAB Function38 ==
  data: chi2_dot output; i input; v input; etam_hat input; delta input; Y_lambda input; chi1 input; R parameter; gamma_lambda parameter
function chi2_dot = fcn(i,v,etam_hat,delta,Y_lambda,chi1, R, gamma_lambda)

chi2_dot = -R*i+v+etam_hat+gamma_lambda*delta*(Y_lambda-delta*chi1);

== matlab function coursework/MATLAB Function39 ==
  data: chi1 input; lambda_hat output; bv input; L parameter; etam_hat input; R parameter
function lambda_hat = fcn(chi1,bv,L,etam_hat, R)

lambda_hat = chi1-L/R*(etam_hat+bv);

== matlab function coursework/MATLAB Function40 ==
  data: chi2_dot output; i input; v input; etam_hat input; delta input; Y_lambda input; chi1 input; R parameter; gamma_lambda parameter
function chi2_dot = fcn(i,v,etam_hat,delta,Y_lambda,chi1, R, gamma_lambda)

chi2_dot = -R*i+v+etam_hat+gamma_lambda*delta*(Y_lambda-delta*chi1);

== matlab function coursework/MATLAB Function41 ==
  data: chi1 input; lambda_hat output; L parameter; etam_hat input; R parameter
function lambda_hat = fcn(chi1,L,etam_hat, R)

lambda_hat = chi1-L/R*(etam_hat);

== matlab function coursework/MATLAB Function3 ==
  data: xi3 input; xi1 input; ym input; xi3_dot output; v parameter; i input; L parameter
function xi3_dot = fcn(xi3,xi1,ym,v,i, L)

xi3_dot = -v*xi3+(ym')*xi1+v^2*L^2*i'*i;

== matlab function coursework/position estimator ==
  settings: updateMethod=DISCRETE
  data: x input; hat_theta output
function hat_theta = angle (x)
%% 
%declare previous atan2 result (it is zero at the start)
persistent atan2_prev;

if (isempty (atan2_prev))
    atan2_prev = 0;
end
%declare previous estimate hat_theta prev (it is zero at the start)
persistent hat_theta_prev;
if (isempty (hat_theta_prev) )
    hat_theta_prev = 0;
end
%The four-quadrant inverse tangent, atan2 (Y,X), returns values in the closed interval [-pi, pi]
atan2_now=atan2(x(2),x(1));
%% increment the result at atan2 boundaries "-pi" and "+pi"
%calculate the difference
Diff_atan2 = atan2_now - atan2_prev;
%check if we have boundary cases
if (Diff_atan2 > pi)
    Diff_atan2 = Diff_atan2 - 2*pi;
elseif (Diff_atan2 < -pi)
    Diff_atan2 = Diff_atan2 + 2*pi;
end
%% calculate new angle pasting together angles at atan2 boundaries
hat_theta = hat_theta_prev + Diff_atan2;
% updating
atan2_prev = atan2_now;
hat_theta_prev = hat_theta;

== matlab function coursework/MATLAB Function4 ==
  data: xi4 input size=[2 1]; xi2 input; xi1 input; xi4_dot output; v parameter
function xi4_dot = fcn(xi4,xi2,xi1,v)

xi4_dot = -v*xi4+v*xi2-xi1;

== matlab function coursework/MATLAB Function5 ==
  data: xi5 input; xi3 input; xi2 input; xi1 input; xi5_dot output; v parameter; i input; ym input; L parameter
function xi5_dot = fcn(xi5,xi3,xi2,xi1,v,i,ym,L)

xi5_dot = -v*xi5+v*xi3-v^2*L^2*i'*i+ym'*(v*xi2-xi1);

== matlab function coursework/MATLAB Function6 ==
  data: xi1 input; FI output size=[2 1]; i input; xi2 input; L parameter; v parameter
function FI = fcn(xi1,i,xi2, L, v)

FI = 2*xi1-2*v*L*i-v*xi2;
